simulink model "H_infinity_augemented_model"  (R2018b)
settings: Solver=FixedStepAuto  StartTime=0.0  StopTime=10  RelTol=1e-3
undefined symbols (not defined in the file): A, A_ob, B, B_ob, C, C2, C_ob, D21, D22, D_ob, den_G, F, K, K_ltr, Ku, Kw, Lu, num_G, P, precomp_stat
libraries: simulink x7
settings Model: Creator=牟城志  LastModifiedBy=牟城志
settings OptimizationCC: DefaultParameterBehavior=Inlined  UseDivisionForNetSlopeComputation=on  UseFloatMulNetSlope=on  InlineInvariantSignals=on  PassReuseOutputArgsAs=Individual arguments  ZeroExternalMemoryAtStartup=off  ZeroInternalMemoryAtStartup=off  NoFixptDivByZeroProtection=on  EfficientFloat2IntCast=on  LifeSpan=1  OptimizeBlockOrder=speed  DifferentSizesBufferReuse=on
settings DebuggingCC: ParameterTunabilityLossMsg=error
settings HardwareCC: ProdLongLongMode=on
settings SFSimCC: MATLABDynamicMemAlloc=off
settings RTWCC: SystemTargetFile=ert.tlc  TemplateMakefile=ert_default_tmf  GenerateReport=on  IncludeHyperlinkInReport=on  LaunchReport=on  GenerateTraceInfo=on  GenerateTraceReport=on  GenerateTraceReportSl=on  GenerateTraceReportSf=on  GenerateTraceReportEml=on  GenerateCodeMetricsReport=on
settings CodeAppCC: ForceParamTrailComments=on  IgnoreCustomStorageClasses=off  OperatorAnnotations=on  SimulinkDataObjDesc=on  SFDataObjDesc=on  CustomSymbolStrGlobalVar=rt$N$M  CustomSymbolStrType=$N$M  CustomSymbolStrFcn=$N$M$F  CustomSymbolStrMacro=$N$M  InsertBlockDesc=on
settings ERTTargetCC: TargetLangStandard=C99 (ISO)  GenerateSampleERTMain=on  IncludeMdlTerminateFcn=off  CombineSignalStateStructs=on  SupportComplex=off  SupportContinuousTime=on  InlinedParameterPlacement=NonHierarchical  ERTCustomFileTemplate=example_file_process.tlc  ERTFilePackagingFormat=CompactWithDataFile

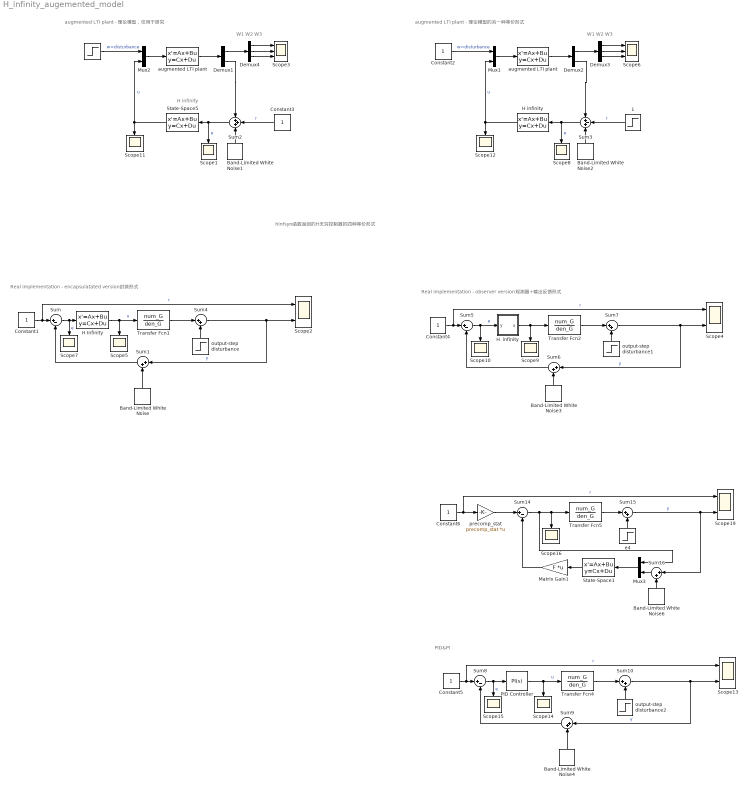
== system H_infinity_augemented_model ==
  note: hinfsyn函数返回的H无穷控制器的四种等价形式
  note: H infinity
  note: augmented LTI plant - 理论模型，仅用于研究
  note: Real implementation - encapsulatated version 封装形式
  note: W1 W2 W3
  note: augmented LTI plant - 理论模型的另一种等价形式
  note: W1 W2 W3
  note: Real implementation - observer version 观测器+输出反馈形式
  note: PID&PI
  " " : Step  Time=4  After=-0.5  SampleTime=0
  " 1" : Step  Time=4  After=0.5  SampleTime=0
  " H infinity" : StateSpace  A=K.A  B=K.B  C=K.C  D=K.D  InitialCondition=0
  " e4" : Step  Time=4  After=0.5  SampleTime=0
  Band-Limited White Noise{,1..4,6} (6 alike) : simulink/Sources/Band-Limited White Noise  Cov=1e-7  Ts=1e-3  seed=[23341]
  Constant{1..6} (6 alike) : Constant
  Demux1 : Demux  Outputs=2
  Demux2 : Demux  Outputs=2
  Demux3 : Demux  Outputs=3
  Demux4 : Demux  Outputs=3
  H  infinity : Subsystem
  H Infinity : StateSpace  A=K.A  B=K.B  C=K.C  D=K.D  InitialCondition=0
  Matrix Gain1 : Gain  Gain=F  Multiplication=Matrix(K*u)  SaturateOnIntegerOverflow=on  OutDataTypeStr=Inherit: Same as input  ParamDataTypeStr=Inherit: Same as input
  Mux1 : Mux  Inputs=2
  Mux2 : Mux  Inputs=2
  Mux3 : Mux  Inputs=2
  PID Controller : simulink/Continuous/PID Controller  Controller=PI  Form=Parallel  TimeDomain=Continuous-time  SampleTime=-1  IntegratorMethod=Forward Euler  FilterMethod=Forward Euler  ControllerParametersSource=internal  P=0.0476550393835022  I=0.882488856497483  D=9.17335238895913  UseFilter=on  N=1154.55051341775  TunerSelectOption=Transfer Function Based (PID Tuner App)  InitialConditionSource=internal  InitialConditionForIntegrator=0  InitialConditionForFilter=0  DifferentiatorICPrevScaledInput=0  ExternalReset=none  TrackingMode=off  Kt=1  LimitOutput=off  UpperSaturationLimit=inf  LowerSaturationLimit=-inf  LinearizeAsGain=on  AntiWindupMode=none  Kb=1  POutMin=[]  POutMax=[]  IOutMin=[]  IOutMax=[]  DOutMin=[]  DOutMax=[]  NOutMin=[]  NOutMax=[]  SumOutMin=[]  SumOutMax=[]  SaturationOutMin=[]  SaturationOutMax=[]  PParamMin=[]  PParamMax=[]  IParamMin=[]  IParamMax=[]  DParamMin=[]  DParamMax=[]  NParamMin=[]  NParamMax=[]  KbParamMin=[]  KbParamMax=[]  KtParamMin=[]  KtParamMax=[]  KbOutMin=[]  KbOutMax=[]  KtOutMin=[]  KtOutMax=[]  IntegratorOutMin=[]  IntegratorOutMax=[]  FilterOutMin=[]  FilterOutMax=[]  SumI1OutMin=[]  SumI1OutMax=[]  SumI2OutMin=[]  SumI2OutMax=[]  SumI3OutMin=[]  SumI3OutMax=[]  SumI4OutMin=[]  SumI4OutMax=[]  SumDOutMin=[]  SumDOutMax=[]  DifferentiatorOutMin=[]  DifferentiatorOutMax=[]  FilterDiffOutCoefMin=[]  FilterDiffOutCoefMax=[]  ReciprocalOutMin=[]  ReciprocalOutMax=[]  SumDenOutMin=[]  SumDenOutMax=[]  SumNumOutMin=[]  SumNumOutMax=[]  DivideOutMin=[]  DivideOutMax=[]  IntegratorContinuousStateAttributes=''  IntegratorStateMustResolveToSignalObject=off  IntegratorRTWStateStorageClass=Auto  FilterContinuousStateAttributes=''  FilterStateMustResolveToSignalObject=off  FilterRTWStateStorageClass=Auto  ParallelPVariant=InternalParameters  IdealPVariant=Disabled  IVariant=InternalParameters  DVariant=Disabled  IntegratorVariant=Continuous  SatVariant=Disabled  AWVariant=Passthrough  PCopyVariant=Disabled  TRVariant=Disabled  FdbkBlocksVariant=Forward  IdealPFdbkVariant=Disabled  SatFdbkVariant=Disabled  DerivativeFilterVariant=Disabled  NVariant=Disabled  NCopyVariant=Disabled_SignalSpec  FilterICVariant=Disabled  IntegratorICVariant=InternalICs  ExternalResetVariant=Disabled  TRSumVariant=Passthrough  SumFdbkVariant=Disabled  SumVariant=Sum_PI
  Scope{1,5,7..12,14..16} (11 alike) : Scope
  Scope{2,4,13,19} (4 alike) : Scope  NumInputPorts=2
  Scope3 : Scope  NumInputPorts=3
  Scope6 : Scope  NumInputPorts=3
  State-Space1 : StateSpace  A=A-K_ltr*C  B=[B K_ltr]  C=eye(length(A))  D=zeros(2,2)  InitialCondition=0
  State-Space5 : StateSpace  A=K.A  B=K.B  C=K.C  D=K.D  InitialCondition=0
  Sum : Sum  Inputs=|+-
  Sum{1,4,6..7,9..10} (6 alike) : Sum  Inputs=|++
  Sum14 : Sum  Inputs=|+-  SaturateOnIntegerOverflow=on  InputSameDT=on  OutDataTypeStr=Inherit: Same as first input
  Sum15 : Sum  Inputs=|++  SaturateOnIntegerOverflow=on  InputSameDT=on  OutDataTypeStr=Inherit: Same as first input
  Sum16 : Sum  Inputs=|++  SaturateOnIntegerOverflow=on  InputSameDT=on  OutDataTypeStr=Inherit: Same as first input
  Sum2 : Sum  Inputs=+++
  Sum3 : Sum  Inputs=+-+
  Sum5 : Sum  Inputs=|+-
  Sum8 : Sum  Inputs=|+-
  Transfer Fcn{1..2,4..5} (4 alike) : TransferFcn  Numerator=num_G  Denominator=den_G
  augmented LTI plant : StateSpace  A=P.A  B=P.B  C=P.C  D=P.D  InitialCondition=[0 0 0]
  "augmented LTI plant " : StateSpace  A=P.A  B=P.B  C=P.C  D=P.D  InitialCondition=[0 0 0]
  output-step disturbance : Step  Time=4  After=0.5  SampleTime=0
  output-step disturbance1 : Step  Time=4  After=0.5  SampleTime=0
  output-step disturbance2 : Step  Time=4  After=0.5  SampleTime=0
  precomp_stat : Gain  Gain=precomp_stat  Multiplication=Matrix(K*u)  SaturateOnIntegerOverflow=on  OutDataTypeStr=Inherit: Same as input  ParamDataTypeStr=Inherit: Same as input
  wires:
  Transfer Fcn1/1 -> Sum4/1
  Sum1/1 -> Sum/2
  H Infinity/1 -> Scope5/1, Transfer Fcn1/1  "u"
  Constant1/1 -> Scope2/1, Sum/1  "r"
  Sum/1 -> Scope7/1, H Infinity/1  "e"
  Sum4/1 -> Scope2/2, Sum1/1  "y"
  Constant3/1 -> Sum2/2  "r"
  Band-Limited White Noise1/1 -> Sum2/3
  Sum2/1 -> Scope1/1, State-Space5/1  "e"
  Demux4/3 -> Scope3/3
  Demux4/2 -> Scope3/2
  Demux1/1 -> Demux4/1
  Demux4/1 -> Scope3/1
  State-Space5/1 -> Scope11/1, Mux2/2  "u"
  Demux1/2 -> Sum2/1
  augmented LTI plant/1 -> Demux1/1
  " "/1 -> Mux2/1  "w=disturbance"
  Mux2/1 -> augmented LTI plant/1
  Mux1/1 -> "augmented LTI plant "/1
  Constant2/1 -> Mux1/1  "w=disturbance"
  "augmented LTI plant "/1 -> Demux2/1
  Demux2/2 -> Sum3/1
  " H infinity"/1 -> Mux1/2, Scope12/1  "u"
  Demux3/1 -> Scope6/1
  Demux2/1 -> Demux3/1
  Demux3/2 -> Scope6/2
  Demux3/3 -> Scope6/3
  Sum3/1 -> Scope8/1, " H infinity"/1  "e"
  Band-Limited White Noise2/1 -> Sum3/3
  " 1"/1 -> Sum3/2  "r"
  Sum7/1 -> Scope4/2, Sum6/1  "y"
  Sum5/1 -> H  infinity/1(y), Scope10/1  "e"
  Constant4/1 -> Sum5/1, Scope4/1  "r"
  Sum6/1 -> Sum5/2
  Transfer Fcn2/1 -> Sum7/1
  output-step disturbance1/1 -> Sum7/2
  Band-Limited White Noise3/1 -> Sum6/2
  H  infinity/1(u) -> Scope9/1, Transfer Fcn2/1
  output-step disturbance/1 -> Sum4/2
  Band-Limited White Noise/1 -> Sum1/2
  Band-Limited White Noise4/1 -> Sum9/2
  output-step disturbance2/1 -> Sum10/2
  Sum10/1 -> Sum9/1, Scope13/2  "y"
  Sum8/1 -> Scope15/1, PID Controller/1  "e"
  Constant5/1 -> Sum8/1, Scope13/1  "r"
  PID Controller/1 -> Transfer Fcn4/1, Scope14/1  "u"
  Sum9/1 -> Sum8/2
  Transfer Fcn4/1 -> Sum10/1
  Matrix Gain1/1 -> Sum14/2
  Sum14/1 -> Transfer Fcn5/1, Scope16/1, Mux3/1
  State-Space1/1 -> Matrix Gain1/1
  Transfer Fcn5/1 -> Sum15/1
  " e4"/1 -> Sum15/2
  Mux3/1 -> State-Space1/1
  precomp_stat/1 -> Sum14/1
  Sum16/1 -> Mux3/2
  Band-Limited White Noise6/1 -> Sum16/2
  Sum15/1 -> Scope19/2, Sum16/1  "y"
  Constant6/1 -> Scope19/1, precomp_stat/1  "r"

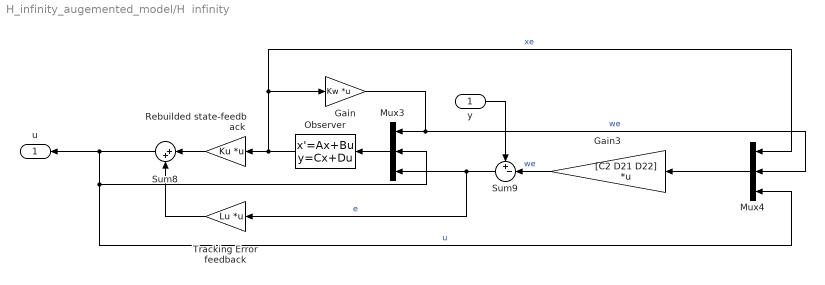
== system H_infinity_augemented_model/H  infinity ==
  y : Inport
  Gain : Gain  Gain=Kw  Multiplication=Matrix(K*u)
  Gain3 : Gain  Gain=[C2 D21 D22]  Multiplication=Matrix(K*u)
  Mux3 : Mux  Inputs=3
  Mux4 : Mux  Inputs=3
  Observer : StateSpace  A=A_ob  B=B_ob  C=C_ob  D=D_ob  InitialCondition=0
  Rebuilded state-feedback : Gain  Gain=Ku  Multiplication=Matrix(K*u)
  Sum8 : Sum  Inputs=|++
  Sum9 : Sum  Inputs=+-|
  Tracking Error feedback : Gain  Gain=Lu  Multiplication=Matrix(K*u)
  u : Outport
  wires:
  Rebuilded state-feedback/1 -> Sum8/1
  Sum8/1 -> u/1, Mux4/3, Mux3/2  "u"
  Tracking Error feedback/1 -> Sum8/2
  Gain/1 -> Mux4/2, Mux3/1  "we"
  Observer/1 -> Rebuilded state-feedback/1, Gain/1, Mux4/1  "xe"
  Mux3/1 -> Observer/1
  Sum9/1 -> Tracking Error feedback/1, Mux3/3  "e"
  Gain3/1 -> Sum9/2  "we"
  Mux4/1 -> Gain3/1
  y/1 -> Sum9/1
